simulink model "Week2_prob4"  (R2020b)
settings: Solver=VariableStepAuto  StartTime=0.0  StopTime=10.0  RelTol=1e-3
undefined symbols (not defined in the file or in its folder): b, J, K, L, R
settings Model: Creator=Lakshmi  LastModifiedBy=Lakshmi

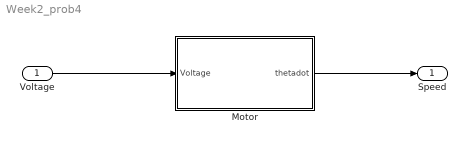
== system Week2_prob4 ==
  Voltage : Inport
  Motor : Subsystem
  Speed : Outport
  wires:
  Motor/1(thetadot) -> Speed/1
  Voltage/1 -> Motor/1(Voltage)

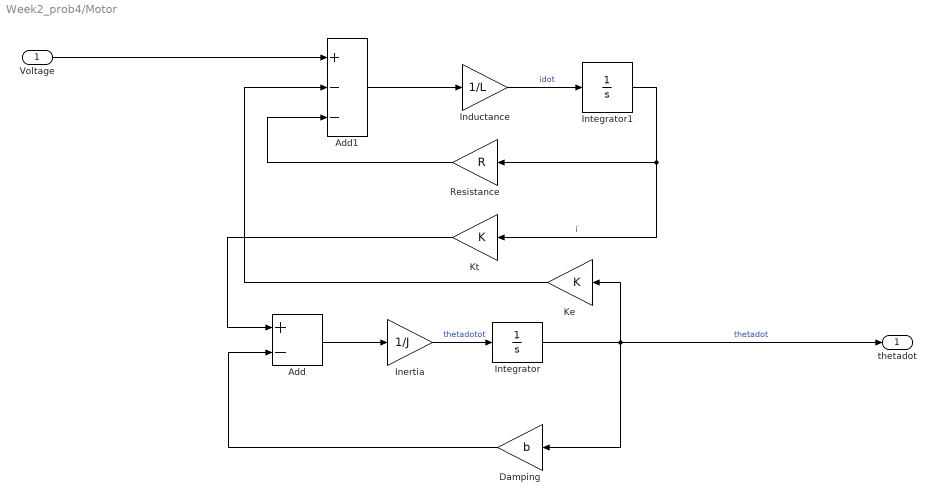
== system Week2_prob4/Motor ==
  Voltage : Inport
  Add : Sum  Inputs=+-
  Add1 : Sum  Inputs=+--
  Damping : Gain  Gain=b
  Inductance : Gain  Gain=1/L
  Inertia : Gain  Gain=1/J
  Integrator : Integrator
  Integrator1 : Integrator
  Ke : Gain  Gain=K
  Kt : Gain  Gain=K
  Resistance : Gain  Gain=R
  thetadot : Outport
  wires:
  Integrator1/1 -> Kt/1, Resistance/1  "i"
  Kt/1 -> Add/1
  Inductance/1 -> Integrator1/1  "idot"
  Damping/1 -> Add/2
  Inertia/1 -> Integrator/1  "thetadotot"
  Integrator/1 -> thetadot/1, Ke/1, Damping/1  "thetadot"
  Add1/1 -> Inductance/1
  Add/1 -> Inertia/1
  Voltage/1 -> Add1/1
  Resistance/1 -> Add1/3
  Ke/1 -> Add1/2
